simulink model "SYNGEN"  (Simulink 7.5)
settings: Solver=ode23  StartTime=0.0  StopTime=600.0  FixedStep=0.01  MaxStep=0.05  MinStep=0.0001  RelTol=1
libraries: simulink x1
settings Model: Creator=avnish  LastModifiedBy=avnish
settings SolverCC: InitialStep=0.02
settings DataIOCC: SignalLoggingName=sigsOut
settings OptimizationCC: BlockReduction=off  BooleanDataType=off
settings DebuggingCC: SaveWithParameterizedLinksMsg=none  SignalResolutionControl=TryResolveAllWithWarning  SolverPrmCheckMsg=none  MultiTaskDSMMsg=warning  MultiTaskCondExecSysMsg=none  StrictBusMsg=None
settings HardwareCC: TargetUnknown=on
settings RTWCC: IncludeERTFirstTime=on

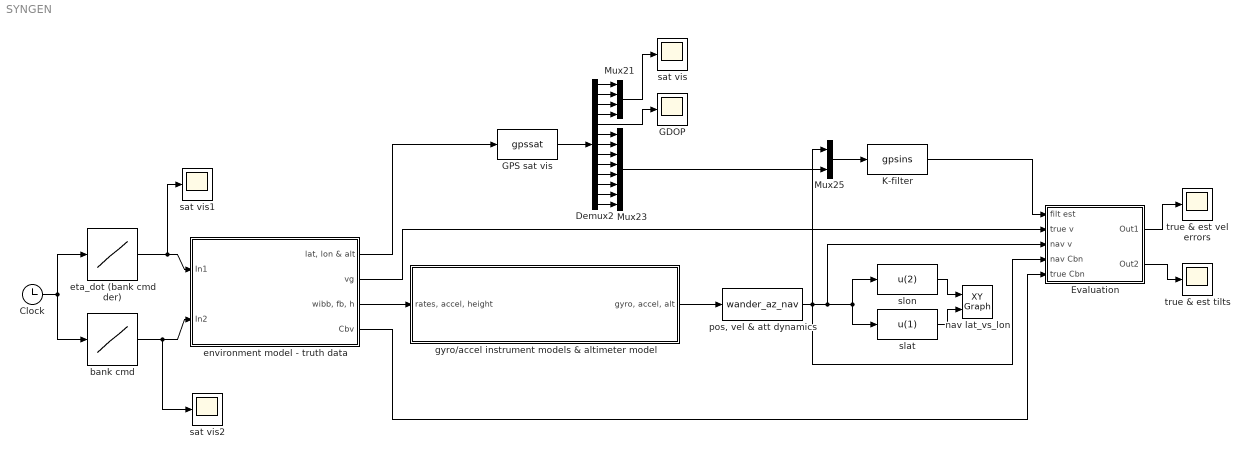
== system SYNGEN ==
  Clock : Clock
  Demux2 : Demux  Outputs=13
  Evaluation : Subsystem
  GDOP : Scope
      settings: YMin=3.45  YMax=3.75  SaveName=ScopeData5  MaxDataPoints=60000  Decimation=10
  GPS sat vis : S-Function  FunctionName=gpssat  EnableBusSupport=off
  K-filter : S-Function  FunctionName=gpsins  Parameters=1.0,1000.0^2,1000.0^2,1000.0^2,10.0^2,10.0^2,10.0^2,1.0e-6,1.0e-6,1.0e-6,10.0^2,10.0^2,1.0^2,0,-600.,0  EnableBusSupport=off
  Mux21 : Mux
  Mux23 : Mux  Inputs=8
  Mux25 : Mux  Inputs=2
  "bank cmd " : Lookup  InputValues=[0,60.,70.,90.,100.,160.,170.,190.,200.,260.,270.,290.,300.,360.,370.,390.,400.,600.]  Table=[0,0,25.,25.,0,0,-25.,-25.,0,0,0,0,0,0,0,0,0,0]  OutDataType=sfix(16)  OutScaling=2^0  SaturateOnIntegerOverflow=on
  environment model - truth data : Subsystem
  eta_dot (bank cmd der) : Lookup  InputValues=[0,59.99,60.01,69.99,70.01,89.99,90.01,99.99,100.01,159.99,160.01,169.99,170.01,189.99,190.01,199.99,200.01,259.99,260.01,269.99,270.01,289.99,290.01,299.99,300.01,359.99,360.01,369.99,370.01,389.99,390.01,399.99,400.01,600.]  Table=[0,0,2.5,2.5,0,0,-2.5,-2.5,0,0,-2.5,-2.5,0,0,2.5,2.5,0,0,-0.0,-0.0,0,0,0.0,0.0,0,0,0.0,0.0,0,0,-0.0,-0.0,0,0]  OutDataType=sfix(16)  OutScaling=2^0  SaturateOnIntegerOverflow=on
  gyro/accel instrument models & altimeter model : Subsystem
  nav lat_vs_lon : simulink/Sinks/XY Graph  SystemSampleTime=-1  xmin=-86.8  xmax=-85.6  ymin=30.  ymax=30.8  st=1
  "pos, vel & att dynamics" : S-Function  FunctionName=wander_az_nav  Parameters=-6.17875e-5,1.85093e-4,7.07415e-1,7.06798e-1,0,-600.,0,.8625137,0,.5060338,-.5051947,.0575641,.8610835,-.0291294,-.9983418,.0496498,100.  EnableBusSupport=off
  sat vis : Scope
      settings: TimeRange=600  YMin=10  YMax=45  SaveName=ScopeData4  MaxDataPoints=60000  Decimation=10
  sat vis1 : Scope
      settings: TimeRange=600  YMin=-2.5  YMax=2.5  MaxDataPoints=60000  Decimation=10
  sat vis2 : Scope
      settings: TimeRange=600  YMin=-25  YMax=25  MaxDataPoints=60000  Decimation=10
  slat : Fcn  Expr=u(1)
  slon : Fcn  Expr=u(2)
  true & est tilts : Scope
      settings: TimeRange=600  YMin=-0.0002  YMax=0.0009  SaveName=ScopeData6  MaxDataPoints=60000
  true & est vel errors : Scope
      settings: TimeRange=600  YMax=10  SaveName=ScopeData3  MaxDataPoints=60000  Decimation=100
  wires:
  Clock/1 -> eta_dot (bank cmd der)/1, "bank cmd "/1
  eta_dot (bank cmd der)/1 -> environment model - truth data/1(In1), sat vis1/1
  "pos, vel & att dynamics"/1 -> Mux25/1, slon/1, slat/1, Evaluation/3(nav v), Evaluation/4(nav Cbn)
  "bank cmd "/1 -> environment model - truth data/2(In2), sat vis2/1
  GPS sat vis/1 -> Demux2/1
  Demux2/5 -> GDOP/1
  Demux2/1 -> Mux21/1
  Demux2/2 -> Mux21/2
  Demux2/3 -> Mux21/3
  Demux2/4 -> Mux21/4
  Mux21/1 -> sat vis/1
  Demux2/6 -> Mux23/1
  Demux2/7 -> Mux23/2
  Demux2/9 -> Mux23/4
  Demux2/10 -> Mux23/5
  Demux2/11 -> Mux23/6
  Demux2/12 -> Mux23/7
  Demux2/13 -> Mux23/8
  Demux2/8 -> Mux23/3
  Mux23/1 -> Mux25/2
  Mux25/1 -> K-filter/1
  K-filter/1 -> Evaluation/1(filt est)
  gyro/accel instrument models & altimeter model/1("gyro, accel, alt") -> "pos, vel & att dynamics"/1
  Evaluation/2(Out2) -> true & est tilts/1
  Evaluation/1(Out1) -> true & est vel errors/1
  slon/1 -> nav lat_vs_lon/1
  slat/1 -> nav lat_vs_lon/2
  environment model - truth data/3("wibb, fb, h") -> gyro/accel instrument models & altimeter model/1("rates, accel, height")
  environment model - truth data/1("lat, lon & alt") -> GPS sat vis/1
  environment model - truth data/2(vg) -> Evaluation/2(true v)
  environment model - truth data/4(Cbv) -> Evaluation/5(true Cbn)

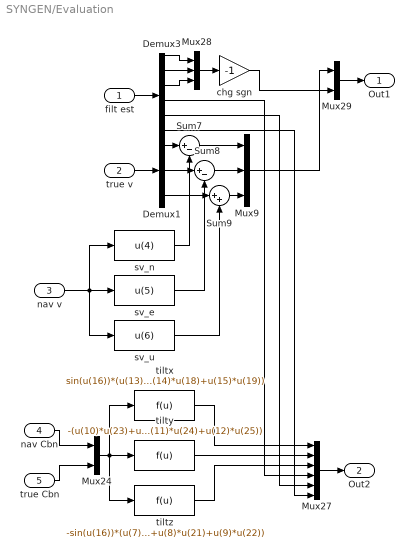
== system SYNGEN/Evaluation ==
  filt est : Inport  OutDataType=sfix(16)  OutScaling=2^0
  true v : Inport  Port=2  OutDataType=sfix(16)  OutScaling=2^0
  nav v : Inport  Port=3  OutDataType=sfix(16)  OutScaling=2^0
  nav Cbn : Inport  Port=4  OutDataType=sfix(16)  OutScaling=2^0
  true Cbn : Inport  Port=5  OutDataType=sfix(16)  OutScaling=2^0
  Demux1 : Demux  Outputs=3
  Demux3 : Demux  Outputs=6
  Mux24 : Mux  Inputs=2
  Mux27 : Mux  Inputs=6
  Mux28 : Mux  Inputs=3
  Mux29 : Mux  Inputs=2
  Mux9 : Mux  Inputs=3
  Sum7 : Sum  Inputs=|+-  OutDataType=sfix(16)  OutScaling=2^0  SaturateOnIntegerOverflow=on  InputSameDT=on  OutDataTypeStr=Inherit: Same as first input
  Sum8 : Sum  Inputs=|+-  OutDataType=sfix(16)  OutScaling=2^0  SaturateOnIntegerOverflow=on  InputSameDT=on  OutDataTypeStr=Inherit: Same as first input
  Sum9 : Sum  Inputs=|++  OutDataType=sfix(16)  OutScaling=2^0  SaturateOnIntegerOverflow=on  InputSameDT=on  OutDataTypeStr=Inherit: Same as first input
  chg sgn : Gain  Gain=-1  ParameterDataType=sfix(16)  ParameterScaling=2^0  OutDataType=sfix(16)  OutScaling=2^0  SaturateOnIntegerOverflow=on  OutDataTypeStr=Inherit: Same as input  ParamDataTypeStr=Inherit: Same as input
  sv_e : Fcn  Expr=u(5)
  sv_n : Fcn  Expr=u(4)
  sv_u : Fcn  Expr=u(6)
  tiltx : Fcn  Expr=sin(u(16))*(u(13)*u(20)+u(14)*u(21)+u(15)*u(22))-cos(u(16))*(u(13)*u(17)+u(14)*u(18)+u(15)*u(19))
  tilty : Fcn  Expr=-(u(10)*u(23)+u(11)*u(24)+u(12)*u(25))
  tiltz : Fcn  Expr=-sin(u(16))*(u(7)*u(17)+u(8)*u(18)+u(9)*u(19))-cos(u(16))*(u(7)*u(20)+u(8)*u(21)+u(9)*u(22))
  Out1 : Outport
  Out2 : Outport  Port=2
  wires:
  sv_n/1 -> Sum7/2
  Demux1/1 -> Sum7/1
  Demux1/2 -> Sum8/1
  sv_e/1 -> Sum8/2
  Sum7/1 -> Mux9/1
  Sum8/1 -> Mux9/2
  Demux1/3 -> Sum9/1
  sv_u/1 -> Sum9/2
  Sum9/1 -> Mux9/3
  Demux3/4 -> Mux27/4
  Demux3/5 -> Mux27/5
  Demux3/6 -> Mux27/6
  Demux3/1 -> Mux28/1
  Demux3/2 -> Mux28/2
  Demux3/3 -> Mux28/3
  Mux28/1 -> chg sgn/1
  Mux24/1 -> tiltz/1, tiltx/1, tilty/1
  tiltx/1 -> Mux27/1
  tilty/1 -> Mux27/2
  tiltz/1 -> Mux27/3
  chg sgn/1 -> Mux29/2
  Mux9/1 -> Mux29/1
  Mux29/1 -> Out1/1
  filt est/1 -> Demux3/1
  true v/1 -> Demux1/1
  nav v/1 -> sv_n/1, sv_e/1, sv_u/1
  nav Cbn/1 -> Mux24/1
  true Cbn/1 -> Mux24/2
  Mux27/1 -> Out2/1

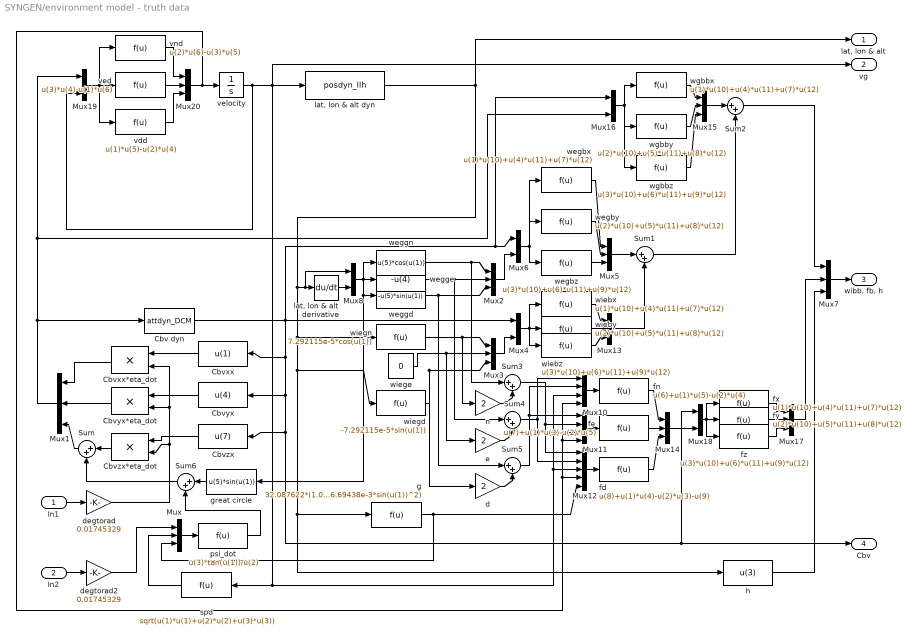
== system SYNGEN/environment model - truth data ==
  In1 : Inport  OutDataType=sfix(16)  OutScaling=2^0
  In2 : Inport  Port=2  OutDataType=sfix(16)  OutScaling=2^0
  Cbv dyn : S-Function  FunctionName=attdyn_DCM  Parameters=0,-1.,0,1.,0.,0,0,0,1.  EnableBusSupport=off
  Cbvxx : Fcn  Expr=u(1)
  Cbvxx*eta_dot : Product  OutDataType=sfix(16)  OutScaling=2^0  SaturateOnIntegerOverflow=on  InputSameDT=on  OutDataTypeStr=Inherit: Same as first input
  Cbvyx : Fcn  Expr=u(4)
  Cbvyx*eta_dot : Product  OutDataType=sfix(16)  OutScaling=2^0  SaturateOnIntegerOverflow=on  InputSameDT=on  OutDataTypeStr=Inherit: Same as first input
  Cbvzx : Fcn  Expr=u(7)
  Cbvzx*eta_dot : Product  OutDataType=sfix(16)  OutScaling=2^0  SaturateOnIntegerOverflow=on  InputSameDT=on  OutDataTypeStr=Inherit: Same as first input
  Mux{,1..3,5,7,13..15,17,20} (11 alike) : Mux  Inputs=3
  Mux10 : Mux
  Mux11 : Mux
  Mux12 : Mux  Inputs=5
  Mux{4,6,8,16,18..19} (6 alike) : Mux  Inputs=2
  Sum{,1..6} (7 alike) : Sum  Inputs=|++  OutDataType=sfix(16)  OutScaling=2^0  SaturateOnIntegerOverflow=on  InputSameDT=on  OutDataTypeStr=Inherit: Same as first input
  d : Gain  Gain=2  ParameterDataType=sfix(16)  ParameterScaling=2^0  OutDataType=sfix(16)  OutScaling=2^0  SaturateOnIntegerOverflow=on  OutDataTypeStr=Inherit: Same as input  ParamDataTypeStr=Inherit: Same as input
  degtorad : Gain  Gain=0.01745329  ParameterDataType=sfix(16)  ParameterScaling=2^0  OutDataType=sfix(16)  OutScaling=2^0  SaturateOnIntegerOverflow=on  OutDataTypeStr=Inherit: Same as input  ParamDataTypeStr=Inherit: Same as input
  degtorad2 : Gain  Gain=0.01745329  ParameterDataType=sfix(16)  ParameterScaling=2^0  OutDataType=sfix(16)  OutScaling=2^0  SaturateOnIntegerOverflow=on  OutDataTypeStr=Inherit: Same as input  ParamDataTypeStr=Inherit: Same as input
  e : Gain  Gain=2  ParameterDataType=sfix(16)  ParameterScaling=2^0  OutDataType=sfix(16)  OutScaling=2^0  SaturateOnIntegerOverflow=on  OutDataTypeStr=Inherit: Same as input  ParamDataTypeStr=Inherit: Same as input
  fd : Fcn  Expr=u(8)+u(1)*u(4)-u(2)*u(3)-u(9)
  fe : Fcn  Expr=u(7)+u(1)*u(3)-u(2)*u(5)
  fn : Fcn  Expr=u(6)+u(1)*u(5)-u(2)*u(4)
  fx : Fcn  Expr=u(1)*u(10)+u(4)*u(11)+u(7)*u(12)
  fy : Fcn  Expr=u(2)*u(10)+u(5)*u(11)+u(8)*u(12)
  fz : Fcn  Expr=u(3)*u(10)+u(6)*u(11)+u(9)*u(12)
  g : Fcn  Expr=32.087622*(1.0+1.93185e-3*sin(u(1))^2)/sqrt(1.0-6.69438e-3*sin(u(1))^2)
  great circle : Fcn  Expr=u(5)*sin(u(1))
  h : Fcn  Expr=u(3)
  "lat, lon & alt derivative" : Derivative
  "lat, lon & alt dyn" : S-Function  FunctionName=posdyn_llh  Parameters=30.4/57.29577951,-86.7/57.2957951,100.0  EnableBusSupport=off
  n : Gain  Gain=2  ParameterDataType=sfix(16)  ParameterScaling=2^0  OutDataType=sfix(16)  OutScaling=2^0  SaturateOnIntegerOverflow=on  OutDataTypeStr=Inherit: Same as input  ParamDataTypeStr=Inherit: Same as input
  psi_dot : Fcn  Expr=u(3)*tan(u(1))/u(2)
  spd : Fcn  Expr=sqrt(u(1)*u(1)+u(2)*u(2)+u(3)*u(3))
  vdd : Fcn  Expr=u(1)*u(5)-u(2)*u(4)
  ved : Fcn  Expr=u(3)*u(4)-u(1)*u(6)
  velocity : Integrator  InitialCondition=[0,600.,0]
  vnd : Fcn  Expr=u(2)*u(6)-u(3)*u(5)
  wegbx : Fcn  Expr=u(1)*u(10)+u(4)*u(11)+u(7)*u(12)
  wegby : Fcn  Expr=u(2)*u(10)+u(5)*u(11)+u(8)*u(12)
  wegbz : Fcn  Expr=u(3)*u(10)+u(6)*u(11)+u(9)*u(12)
  weggd : Fcn  Expr=-u(5)*sin(u(1))
  wegge : Fcn  Expr=-u(4)
  weggn : Fcn  Expr=u(5)*cos(u(1))
  wgbbx : Fcn  Expr=u(1)*u(10)+u(4)*u(11)+u(7)*u(12)
  wgbby : Fcn  Expr=u(2)*u(10)+u(5)*u(11)+u(8)*u(12)
  wgbbz : Fcn  Expr=u(3)*u(10)+u(6)*u(11)+u(9)*u(12)
  wiebx : Fcn  Expr=u(1)*u(10)+u(4)*u(11)+u(7)*u(12)
  wieby : Fcn  Expr=u(2)*u(10)+u(5)*u(11)+u(8)*u(12)
  wiebz : Fcn  Expr=u(3)*u(10)+u(6)*u(11)+u(9)*u(12)
  wiegd : Fcn  Expr=-7.292115e-5*sin(u(1))
  wiege : Constant  Value=0  OutDataType=sfix(16)  OutScaling=2^0
  wiegn : Fcn  Expr=7.292115e-5*cos(u(1))
  "lat, lon & alt" : Outport
  vg : Outport  Port=2
  "wibb, fb, h" : Outport  Port=3
  Cbv : Outport  Port=4
  wires:
  Mux/1 -> psi_dot/1
  Cbv dyn/1 -> Cbvxx/1, Cbvyx/1, Cbvzx/1, Mux18/1, Cbv/1, Mux4/1, Mux6/1, Mux16/1
  Cbvxx/1 -> Cbvxx*eta_dot/1
  Cbvyx/1 -> Cbvyx*eta_dot/1
  Cbvzx/1 -> Cbvzx*eta_dot/1
  Cbvzx*eta_dot/1 -> Sum/1
  Cbvyx*eta_dot/1 -> Mux1/2
  Sum/1 -> Mux1/3
  Cbvxx*eta_dot/1 -> Mux1/1
  Mux1/1 -> Cbv dyn/1, Mux19/1, Mux16/2
  Mux20/1 -> velocity/1, Mux10/4, Mux11/4, Mux12/4
  "lat, lon & alt dyn"/1 -> wiegn/1, wiegd/1, g/1, h/1, "lat, lon & alt derivative"/1, Mux8/1, "lat, lon & alt"/1
  wieby/1 -> Mux13/2
  wiebx/1 -> Mux13/1
  wiebz/1 -> Mux13/3
  wiege/1 -> Mux3/2, e/1
  wiegn/1 -> Mux3/1, n/1
  wiegd/1 -> Mux3/3, d/1
  Mux3/1 -> Mux4/2
  wegge/1 -> Mux2/2, Sum4/1
  weggn/1 -> Mux2/1, Sum3/1
  weggd/1 -> Mux2/3, Sum5/1
  Mux4/1 -> wiebx/1, wieby/1, wiebz/1
  wegby/1 -> Mux5/2
  wegbx/1 -> Mux5/1
  wegbz/1 -> Mux5/3
  Mux6/1 -> wegbx/1, wegby/1, wegbz/1
  Mux2/1 -> Mux6/2
  e/1 -> Sum4/2
  n/1 -> Sum3/2
  d/1 -> Sum5/2
  Mux10/1 -> fn/1
  Mux11/1 -> fe/1
  Mux12/1 -> fd/1
  fe/1 -> Mux14/2
  fn/1 -> Mux14/1
  fd/1 -> Mux14/3
  Mux13/1 -> Sum1/2
  Mux5/1 -> Sum1/1
  wgbby/1 -> Mux15/2
  wgbbx/1 -> Mux15/1
  wgbbz/1 -> Mux15/3
  Mux16/1 -> wgbbx/1, wgbby/1, wgbbz/1
  Mux15/1 -> Sum2/1
  Sum1/1 -> Sum2/2
  Sum2/1 -> Mux7/1
  Mux14/1 -> Mux18/2
  degtorad/1 -> Cbvzx*eta_dot/2, Cbvyx*eta_dot/2, Cbvxx*eta_dot/2
  g/1 -> Mux/3, Mux12/5
  Sum3/1 -> Mux12/1, Mux11/2
  Sum4/1 -> Mux10/1, Mux12/2
  Sum5/1 -> Mux10/2, Mux11/1
  Mux17/1 -> Mux7/2
  spd/1 -> Mux/2
  "lat, lon & alt derivative"/1 -> Mux8/2
  Mux8/1 -> weggn/1, wegge/1, weggd/1, great circle/1
  Mux19/1 -> ved/1, vnd/1, vdd/1
  ved/1 -> Mux20/2
  vnd/1 -> Mux20/1
  vdd/1 -> Mux20/3
  velocity/1 -> "lat, lon & alt dyn"/1, spd/1, Mux10/3, Mux11/3, Mux12/3, vg/1, Mux19/2
  h/1 -> Mux7/3
  great circle/1 -> Sum6/1
  Sum6/1 -> Sum/2
  psi_dot/1 -> Sum6/2
  degtorad2/1 -> Mux/1
  fy/1 -> Mux17/2
  fx/1 -> Mux17/1
  Mux18/1 -> fx/1, fy/1, fz/1
  fz/1 -> Mux17/3
  Mux7/1 -> "wibb, fb, h"/1
  In1/1 -> degtorad/1
  In2/1 -> degtorad2/1

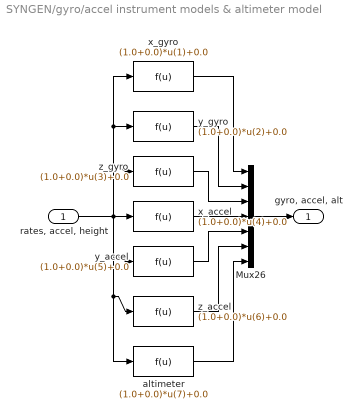
== system SYNGEN/gyro/accel instrument models & altimeter model ==
  "rates, accel, height" : Inport  OutDataType=sfix(16)  OutScaling=2^0
  Mux26 : Mux  Inputs=7
  altimeter : Fcn  Expr=(1.0+0.0)*u(7)+0.0
  x_accel : Fcn  Expr=(1.0+0.0)*u(4)+0.0
  x_gyro : Fcn  Expr=(1.0+0.0)*u(1)+0.0
  y_accel : Fcn  Expr=(1.0+0.0)*u(5)+0.0
  y_gyro : Fcn  Expr=(1.0+0.0)*u(2)+0.0
  z_accel : Fcn  Expr=(1.0+0.0)*u(6)+0.0
  z_gyro : Fcn  Expr=(1.0+0.0)*u(3)+0.0
  "gyro, accel, alt" : Outport
  wires:
  x_accel/1 -> Mux26/4
  y_accel/1 -> Mux26/5
  z_accel/1 -> Mux26/6
  altimeter/1 -> Mux26/7
  z_gyro/1 -> Mux26/3
  y_gyro/1 -> Mux26/2
  x_gyro/1 -> Mux26/1
  "rates, accel, height"/1 -> x_gyro/1, y_gyro/1, z_gyro/1, x_accel/1, y_accel/1, z_accel/1, altimeter/1
  Mux26/1 -> "gyro, accel, alt"/1
